simulink model "Car"  (R2024b)
settings: Solver=ode15s  StartTime=0.0  StopTime=PROFILE_LENGTH  MaxStep=300  RelTol=1e-7
values from neighbouring files (symbols this model uses):
  ACCEL_TOLERANCE = 1    [Setup.m]
  AIR_DENSITY = 1.2    [Setup.m]
  C_ROLLING_RESISTANCE = .0025    (= 0.0025)    [Setup.m]
  CONTROL_MODE = 1    [Setup.m]
  CURRENT_DATA_ECO = ECO_DATA(:, 1)    [Setup.m]
  CURRENT_DATA_POWER = POWER_DATA(:, 1)    [Setup.m]
  D_POWER = 1    [Setup.m]
  D_SPEED = 40    [Setup.m]
  DRAG_COEFFICIENT = 0.25    [Setup.m]
  DRIVER_DISPLAY_DRAW = 2.5    [Setup.m]
  FAN_DRAW = 4.8    [Setup.m]
  FORECASTED_IRRADIANCE = -5*((SOLAR_TIME_BREAKPOINTS-START_TIME).*(SOLAR_TIME_BREAKPOINTS-END_TIME) / (PROFILE_LENGTH/2)^2)    [Setup.m]
  FRONTAL_AREA = 1    [Setup.m]
  FULL_PACK_KWH = HV_PACK_VOLTAGE * HV_PACK_CAPACITY * UNIT_TO_KILO    (= 7.68)    [Setup.m]
  GRAVITY = 9.81    [Setup.m]
  HEADLIGHT_DRAW = 2    [Setup.m]
  HV_PACK_VOLTAGE = 96    [Setup.m]
  I_POWER = 1    [Setup.m]
  I_SPEED = 3    [Setup.m]
  INT_DISTANCES = COURSE_DATA(:, 8) / UNIT_TO_KILO    [Setup.m]
  INT_GRADE_ANGLE = rad2deg(atan(COURSE_DATA(:, 7)/100))    [Setup.m]
  MAX_CURRENT_ECO = max(CURRENT_DATA_ECO)    [Setup.m]
  MAX_CURRENTS_ECO = flip(CURRENT_DATA_ECO)    [Setup.m]
  MAX_CURRENTS_POWER = flip(CURRENT_DATA_POWER)    [Setup.m]
  P_POWER = 10    [Setup.m]
  P_SPEED = 25    [Setup.m]
  REGEN_ON = 0    [Setup.m]
  RPM_BREAKPOINTS_ECO = flip(RPM_DATA_ECO)    [Setup.m]
  RPM_BREAKPOINTS_POWER = flip(RPM_DATA_POWER)    [Setup.m]
  RPM_DATA_ECO = ECO_DATA(:, 3)    [Setup.m]
  RPM_DATA_POWER = POWER_DATA(:, 3)    [Setup.m]
  SECONDS_PER_HOUR = 3600    [Setup.m]
  SOLAR_TIME_BREAKPOINTS = START_TIME:900:END_TIME    [Setup.m]
  SPEED_TO_RPM = 60 / (WHEEL_DIAMETER_METERS * pi)    (= 34.1778689532)    [Setup.m]
  START_TIME = CURRENT_TIME    [Setup.m]
  STARTING_KWH = FULL_PACK_KWH * (1 - 0)    (= 7.68)    [Setup.m]
  TARGET_POWER = 700    [Setup.m]
  TARGET_SPEED = 12    [Setup.m]
  TORQUES_DATA_ECO = ECO_DATA(:, 2)    [Setup.m]
  TORQUES_DATA_POWER = POWER_DATA(:, 2) * 2.5    [Setup.m]
  TOTAL_MASS = CAR_MASS + DRIVER_MASS    (= 282.996279643)    [Setup.m]
  UNIT_TO_KILO = 1 / 1000    (= 0.001)    [Setup.m]
  WHEEL_RADIUS = WHEEL_DIAMETER_METERS / 2    (= 0.2794)    [Setup.m]
undefined symbols (not defined in the file or in its folder): density, density_elevation, distance, elevation, INT_CURRENTS, INT_TORQUES_ECO, MAX_TORQUE
libraries: slpidlib x4, simulink x1
(part 1 of 2)
settings Model: SimulationMode=accelerator  Creator=jcpetrie  LastModifiedBy=luoog
settings ModelReferenceCC: EnableRefExpFcnMdlSchedulingChecks=on
settings RTWCC: GPUComputeCapability=3.5

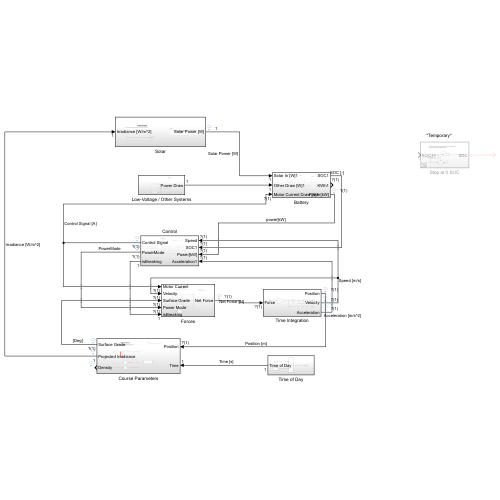
[thumbnail: Simulink's stored preview of the top-level diagram]
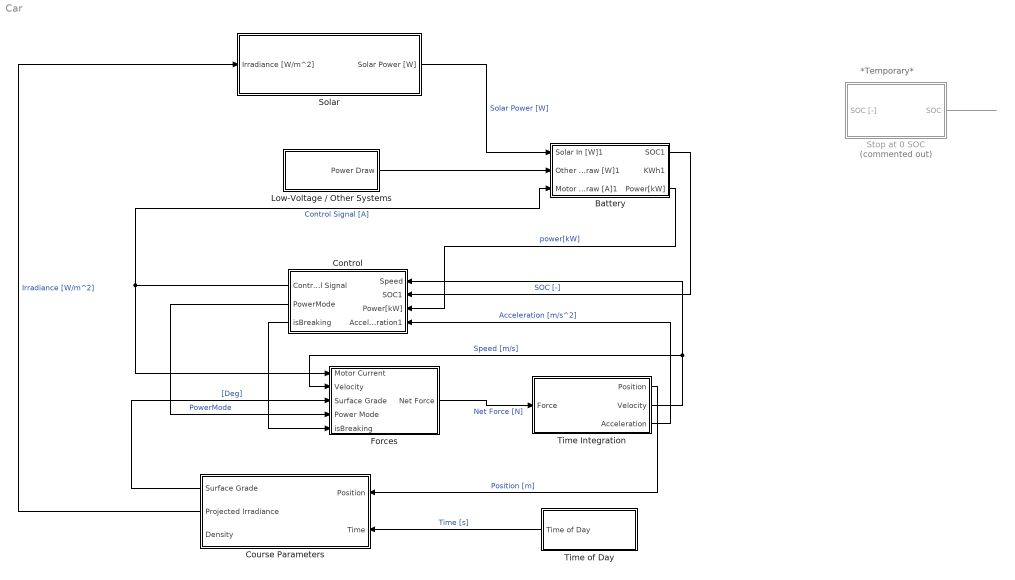
== system Car ==
  note: *Temporary*
  Battery : Subsystem
  Control : Subsystem
  Course Parameters : Subsystem
  Forces : Subsystem
  Low-Voltage / Other Systems : Subsystem
  Solar : Subsystem
  Stop at 0 SOC : Subsystem  Commented=on
  Time Integration : Subsystem
  Time of Day : Subsystem
  wires:
  Control/1(Control Signal) -> Forces/1(Motor Current), Battery/3(Motor Current Draw [A]1)  "Control Signal [A]"
  Time Integration/2(Velocity) -> Control/1(Speed), Forces/2(Velocity)  "Speed [m/s]"
  Forces/1(Net Force) -> Time Integration/1(Force)  "Net Force [N]"
  Time Integration/1(Position) -> Course Parameters/1(Position)  "Position [m]"
  Time Integration/3(Acceleration) -> Control/4(Acceleration1)  "Acceleration [m/s^2]"
  Battery/1(SOC1) -> Control/2(SOC1)  "SOC [-]"
  Course Parameters/1(Surface Grade) -> Forces/3(Surface Grade)  "[Deg]"
  Time of Day/1(Time of Day) -> Course Parameters/2(Time)  "Time [s]"
  Low-Voltage / Other Systems/1(Power Draw) -> Battery/2(Other Draw [W]1)
  Solar/1(Solar Power [W]) -> Battery/1(Solar In [W]1)  "Solar Power [W]"
  Course Parameters/2(Projected Irradiance) -> Solar/1(Irradiance [W/m^2])  "Irradiance [W/m^2]"
  Stop at 0 SOC/1(SOC) -> ?
  Control/2(PowerMode) -> Forces/4(Power Mode)  "PowerMode"
  Battery/3(Power[kW]) -> Control/3(Power[kW])  "power[kW]"
  Control/3(isBreaking) -> Forces/5(isBreaking)

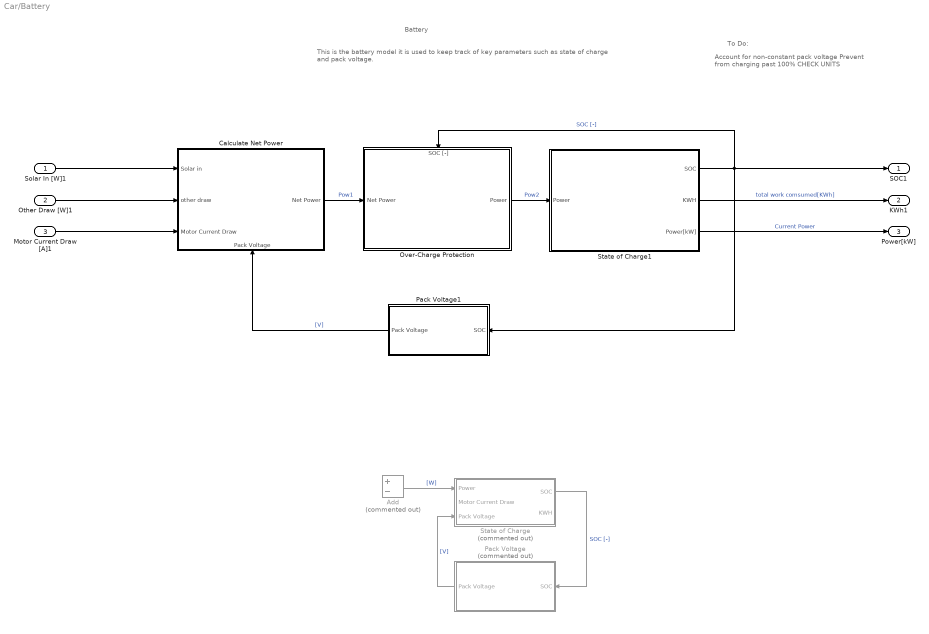
== system Car/Battery ==
  note: To Do:
  note: Battery
  note: This is the battery model it is used to keep track of key parameters such as state of charge and pack voltage.
  note: Account for non-constant pack voltage
      | Prevent from charging past 100%
      | CHECK UNITS
  Solar In [W]1 : Inport
  Other Draw [W]1 : Inport  Port=2
  Motor Current Draw [A]1 : Inport  Port=3
  Add : Sum  Commented=on  Inputs=+-
  Calculate Net Power : Subsystem
      settings: PortSchema="{\"entries\":[{\"content\":{\"sides\":[{\"content\":{\"connectorIds\":[\"In1\",\"In2\",\"In3\"]},\"type\":\"ConnectorPlacement.EquallySpacedRectSide\",\"uuid\":\"e2d2fa73-115a-40a5-bea4-fb1b26f60a86\"},{\"content\":{\"connectorIds\":[\"Out1\"],\"side\":\"RIGHT\"},\"type\":\"ConnectorPlacement.EquallySpacedRectSide\",\"uuid\":\"335f4958-33fa-4255-a87e-d106c2a4918a\"},{\"content\":{\"side\":\"TOP\"},\"type\":\"ConnectorPlacement.EquallySpacedRectSide\",\"uuid\":\"26642419-6030-44a7-8261-db287cf2270e\"},{\"content\":{\"connectorIds\":[\"In4\"],\"side\":\"BOTTOM\"},\"type\":\"ConnectorPlacement.EquallySpacedRectSide\",\"uuid\":\"d53dd7d0-088a-4c9e-b08b-c273ee7e07d3\"}]},\"type\":\"ConnectorPlacement.EquallySpacedConnector\",\"uuid\":\"42977d53-f442-47db-8063-79accecc7adb\"}],\"packageUris\":[\"http://schema.mathworks.com/mf0/Connector/R2020b\"],\"version\":\"1.0\"}"
  Over-Charge Protection : Subsystem
      settings: PortSchema="{\"entries\":[{\"content\":{\"sides\":[{\"content\":{\"connectorIds\":[\"In1\"]},\"type\":\"ConnectorPlacement.EquallySpacedRectSide\",\"uuid\":\"1fd324fe-6fd8-4ed1-a4cf-cd3bc9d77a53\"},{\"content\":{\"connectorIds\":[\"Out1\"],\"side\":\"RIGHT\"},\"type\":\"ConnectorPlacement.EquallySpacedRectSide\",\"uuid\":\"bec321c3-fba2-4d2c-8de0-ad4890ffe26d\"},{\"content\":{\"connectorIds\":[\"In2\"],\"side\":\"TOP\"},\"type\":\"ConnectorPlacement.EquallySpacedRectSide\",\"uuid\":\"f35092d8-5394-4c70-b61a-60d5076cf1ad\"}]},\"type\":\"ConnectorPlacement.EquallySpacedConnector\",\"uuid\":\"3315ea1d-8e02-4ec7-b1c7-14a34191fa6e\"}],\"packageUris\":[\"http://schema.mathworks.com/mf0/Connector/R2020b\"],\"version\":\"1.0\"}"
  Pack Voltage : Subsystem  Commented=on
  Pack Voltage1 : Subsystem
  State of Charge : Subsystem  Commented=on
  State of Charge1 : Subsystem
  SOC1 : Outport
  KWh1 : Outport  Port=2
  Power[kW] : Outport  Port=3
  wires:
  State of Charge/1(SOC) -> Pack Voltage/1(SOC)  "SOC [-]"
  Pack Voltage/1(Pack Voltage) -> State of Charge/3(Pack Voltage)  "[V]"
  Add/1 -> State of Charge/1("Power ")  "[W]"
  State of Charge1/2(KWH) -> KWh1/1  "total work comsumed[KWh]"
  Over-Charge Protection/1(Power) -> State of Charge1/1("Power ")  "Pow2"
  State of Charge1/3(Power[kW]) -> Power[kW]/1  "Current Power"
  Other Draw [W]1/1 -> Calculate Net Power/2(other draw)
  Solar In [W]1/1 -> Calculate Net Power/1(Solar in)
  Motor Current Draw [A]1/1 -> Calculate Net Power/3(Motor Current Draw)
  State of Charge1/1(SOC) -> Pack Voltage1/1(SOC), SOC1/1, Over-Charge Protection/2(SOC [-])  "SOC [-]"
  Calculate Net Power/1(Net Power) -> Over-Charge Protection/1(Net Power)  "Pow1"
  Pack Voltage1/1(Pack Voltage) -> Calculate Net Power/4(Pack Voltage)  "[V]"

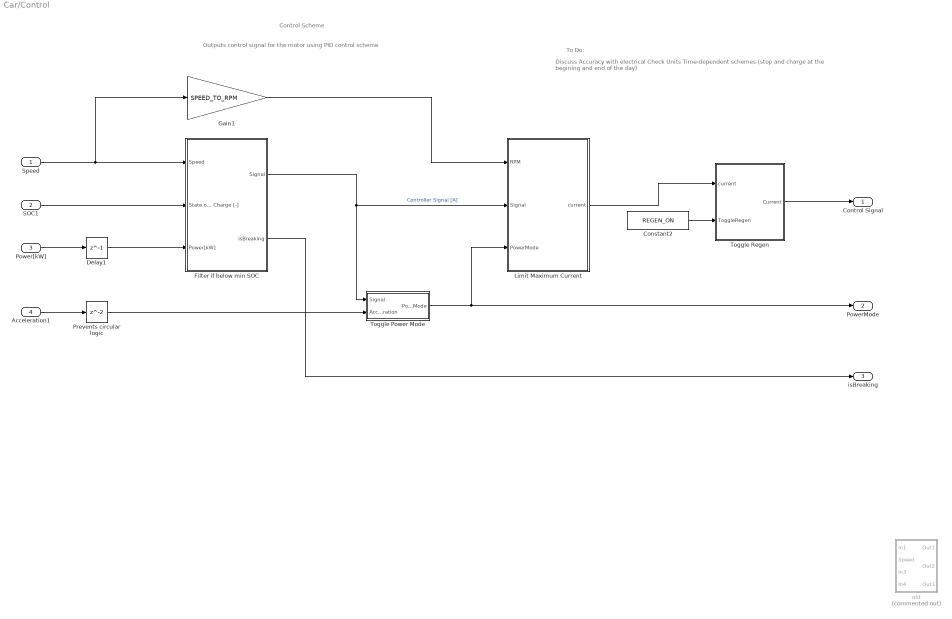
== system Car/Control ==
  note: Outputs control signal for the motor using PID control scheme
  note: To Do:
  note: Control Scheme
  note: Discuss Accuracy with electrical
      | Check Units
      | Time-dependent schemes (stop and charge at the begining and end of the day)
  Speed : Inport
  SOC1 : Inport  Port=2
  Power[kW] : Inport  Port=3
  Acceleration1 : Inport  Port=4
  Constant2 : Constant  Value=REGEN_ON
  Delay1 : Delay  DelayLength=1  SampleTime=5
  Filter if below min SOC : Subsystem
  Gain1 : Gain  Gain=SPEED_TO_RPM
  Limit Maximum Current : Subsystem
  Prevents circular logic : Delay
  Toggle Power Mode : Subsystem
  Toggle Regen : Subsystem
  old : Subsystem  Commented=on
  Control Signal : Outport
  PowerMode : Outport  Port=2
  isBreaking : Outport  Port=3
  wires:
  Toggle Power Mode/1(PowerMode) -> PowerMode/1, Limit Maximum Current/3(PowerMode)
  Limit Maximum Current/1(current) -> Toggle Regen/1(current)
  Toggle Regen/1(Current) -> Control Signal/1
  Constant2/1 -> Toggle Regen/2(ToggleRegen)
  Speed/1 -> Gain1/1, Filter if below min SOC/1(Speed)
  Prevents circular logic/1 -> Toggle Power Mode/2(Acceleration)
  SOC1/1 -> Filter if below min SOC/2(State of Charge [-])
  Filter if below min SOC/2(isBreaking) -> isBreaking/1
  Filter if below min SOC/1(Signal) -> Toggle Power Mode/1(Signal), Limit Maximum Current/2(Signal)  "Controller Signal [A]"
  Gain1/1 -> Limit Maximum Current/1(RPM)
  Power[kW]/1 -> Delay1/1
  Acceleration1/1 -> Prevents circular logic/1
  Delay1/1 -> Filter if below min SOC/3(Power[kW])

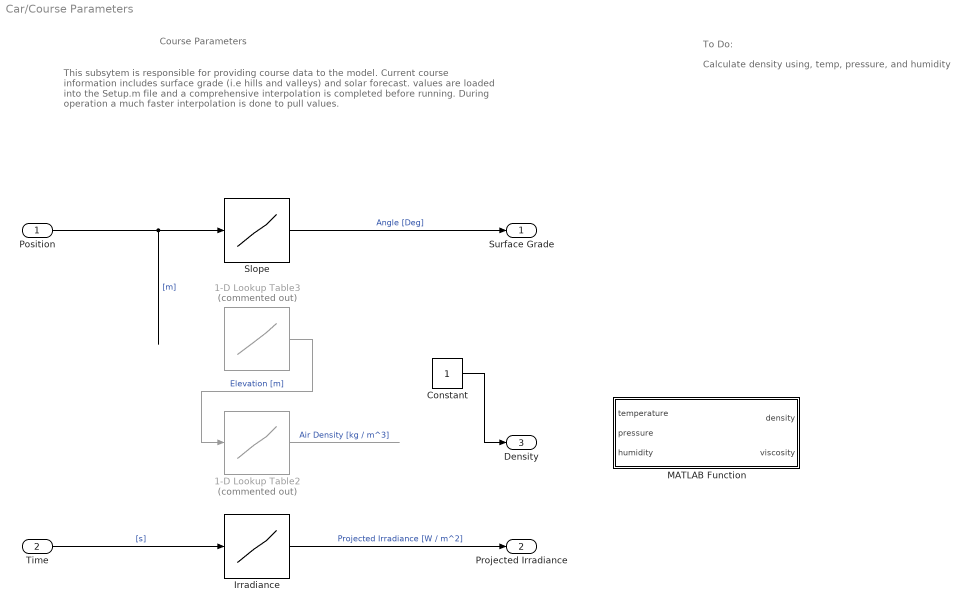
== system Car/Course Parameters ==
  note: Course Parameters
  note: This subsytem is responsible for providing course data to the model. Current course information includes surface grade (i.e hills and valleys) and solar forecast. values are loaded into the Setup.m file and a comprehensive interpolation is completed before running. During operation a much faster interpolation is done to pull values.
  note: To Do:
  note: Calculate density using, temp, pressure, and humidity
  Position : Inport
  Time : Inport  Port=2
  1-D Lookup Table2 : Lookup_n-D  Commented=on  NumberOfTableDimensions=1  BreakpointsForDimension1=density_elevation  Table=density  InternalRulePriority=Speed  RndMeth=Simplest
  1-D Lookup Table3 : Lookup_n-D  Commented=on  NumberOfTableDimensions=1  BreakpointsForDimension1=distance  Table=elevation  InternalRulePriority=Speed  RndMeth=Simplest
  Constant : Constant
  Irradiance : Lookup_n-D  NumberOfTableDimensions=1  BreakpointsForDimension1=SOLAR_TIME_BREAKPOINTS  Table=FORECASTED_IRRADIANCE  InternalRulePriority=Speed  RndMeth=Simplest
  MATLAB Function : MATLAB Function  TreatAsAtomicUnit=on
  Slope : Lookup_n-D  NumberOfTableDimensions=1  BreakpointsForDimension1=INT_DISTANCES  IndexSearchMethod=Linear search  Table=INT_GRADE_ANGLE  ExtrapMethod=Clip  UseLastTableValue=on  InternalRulePriority=Speed  RndMeth=Simplest
  Surface Grade : Outport
  Projected Irradiance : Outport  Port=2
  Density : Outport  Port=3
  wires:
  Position/1 -> Slope/1  "[m]"
  Time/1 -> Irradiance/1  "[s]"
  Slope/1 -> Surface Grade/1  "Angle [Deg]"
  Irradiance/1 -> Projected Irradiance/1  "Projected Irradiance [W / m^2]"
  1-D Lookup Table3/1 -> 1-D Lookup Table2/1  "Elevation [m]"
  1-D Lookup Table2/1 -> ?  "Air Density [kg / m^3]"
  Constant/1 -> Density/1

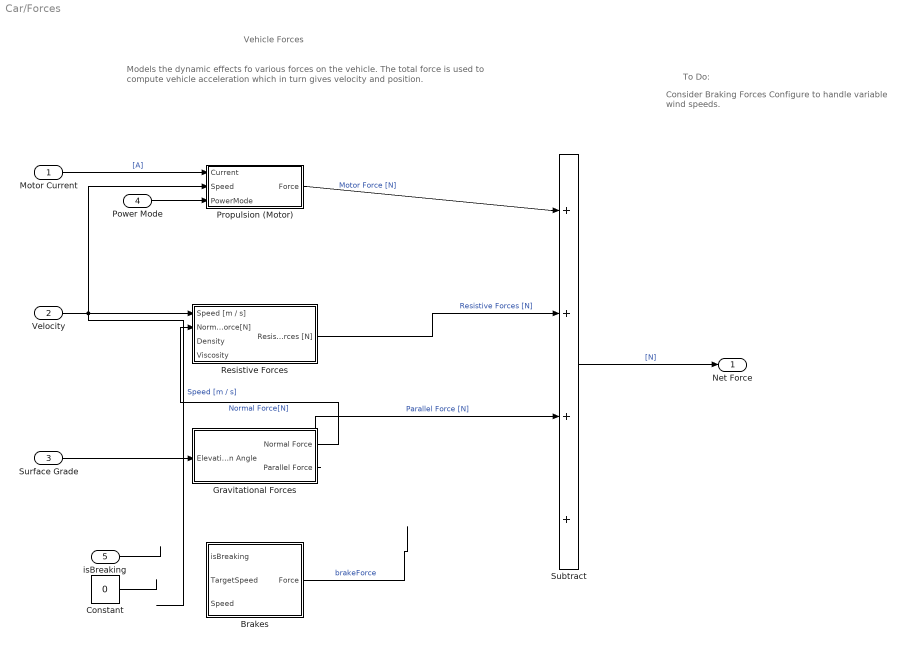
== system Car/Forces ==
  note: To Do:
  note: Vehicle Forces
  note: Models the dynamic effects fo various forces on the vehicle. The total force is used to compute vehicle acceleration which in turn gives velocity and position.
  note: Consider Braking Forces
      | Configure to handle variable wind speeds.
  Motor Current : Inport
  Velocity : Inport  Port=2
  Surface Grade : Inport  Port=3
  Power Mode : Inport  Port=4
  isBreaking : Inport  Port=5
  Brakes : Subsystem
  Constant : Constant  Value=0
  Gravitational Forces : Subsystem
  Propulsion (Motor) : Subsystem
  Resistive Forces : Subsystem
  Subtract : Sum  Inputs=+|+|++
  Net Force : Outport
  wires:
  Propulsion (Motor)/1(Force) -> Subtract/1  "Motor Force [N]"
  Subtract/1 -> Net Force/1  "[N]"
  Motor Current/1 -> Propulsion (Motor)/1(Current)  "[A]"
  Surface Grade/1 -> Gravitational Forces/1(Elevation Angle)
  Gravitational Forces/2(Parallel Force) -> Subtract/3  "Parallel Force [N]"
  Velocity/1 -> Propulsion (Motor)/2(Speed), Resistive Forces/1(Speed [m / s])  "Speed [m / s]"
  Gravitational Forces/1(Normal Force) -> Resistive Forces/2(Normal Force[N])  "Normal Force[N]"
  Resistive Forces/1(Resistive Forces [N]) -> Subtract/2  "Resistive Forces [N]"
  Power Mode/1 -> Propulsion (Motor)/3(PowerMode)
  Constant/1 -> ?
  isBreaking/1 -> ?
  Brakes/1(Force) -> ?  "brakeForce"

== system Car/Low-Voltage // Other Systems ==
  note: Lights
      | Display
      | Raspberry Pi
  Constant1 : Constant  Value=DRIVER_DISPLAY_DRAW
  Constant2 : Constant  Value=HEADLIGHT_DRAW
  Fans : Constant  Value=FAN_DRAW
  Sum : Sum  Inputs=+++
  Power Draw : Outport
  wires:
  Constant1/1 -> Sum/2  "[W]"
  Sum/1 -> Power Draw/1  "[W]"
  Fans/1 -> Sum/1  "[W]"
  Constant2/1 -> Sum/3  "[W]"

== system Car/Solar ==
  note: Remove constant power out
      | Replace with conversion function based on experimental data which converts irradiance to power
  note: Converts expected irradiance to solar out. Based on testing data.
  note: Solar Power
  note: To Do:
  Irradiance [W/m^2] : Inport
  Solar Power [W] : Outport
  wires:
  Irradiance [W/m^2]/1 -> Solar Power [W]/1

== system Car/Stop at 0 SOC ==
  note: This block is a temporary fix meant to adress issues that occor when the car attempts to draw power when the battery is empty.
  SOC [-] : Inport
  If : If
  If Action Subsystem : Subsystem  TreatAsAtomicUnit=on
  If Action Subsystem1 : Subsystem  TreatAsAtomicUnit=on
  Stop Simulation : Stop
  SOC : Outport
  wires:
  If/1 -> If Action Subsystem/Action
  SOC [-]/1 -> If Action Subsystem1/1(SOC), If Action Subsystem/1(SOC), If/1
  If Action Subsystem1/1(Out1) -> Stop Simulation/1
  If/2 -> If Action Subsystem1/Action
  If Action Subsystem/1(Out1) -> SOC/1

== system Car/Time Integration ==
  Force : Inport
  Gain : Gain  Gain=1 / TOTAL_MASS
  Integrator : Integrator
  Integrator1 : Integrator
  Position : Outport
  Velocity : Outport  Port=2
  Acceleration : Outport  Port=3
  wires:
  Gain/1 -> Acceleration/1, Integrator/1  "Acceleration [m/s^2]"
  Integrator/1 -> Velocity/1, Integrator1/1  "Velocity [m/s]"
  Force/1 -> Gain/1  "[N]"
  Integrator1/1 -> Position/1  "Position [m]"

== system Car/Time of Day ==
  Add : Sum
  Clock : Clock
  Constant : Constant  Value=START_TIME
  Time of Day : Outport
  wires:
  Add/1 -> Time of Day/1  "Time of Day [s]"
  Clock/1 -> Add/1  "Simulation Time [s]"
  Constant/1 -> Add/2  "Start time of day [s]"

== system Car/Battery/Calculate Net Power ==
  Solar in : Inport
  other draw : Inport  Port=2
  Motor Current Draw : Inport  Port=3
  Pack Voltage : Inport  Port=4
  Plus : Sum  Inputs=+--
  Product : Product  Inputs=**
  Net Power : Outport
  wires:
  Product/1 -> Plus/3  "[W]"
  Plus/1 -> Net Power/1
  Motor Current Draw/1 -> Product/1  "[A]"
  Pack Voltage/1 -> Product/2  "[V]"
  other draw/1 -> Plus/2
  Solar in/1 -> Plus/1

== system Car/Battery/Over-Charge Protection ==
  Net Power : Inport
  SOC [-] : Inport  Port=2
  Charged status : Merge
  Fully charged : Subsystem  TreatAsAtomicUnit=on
  Not fully charged : Subsystem  TreatAsAtomicUnit=on
  Overcharge Prevention : If  IfExpression=u1 >=MAX_SOC  ZeroCross=off
  Power : Outport
  wires:
  Net Power/1 -> Fully charged/1(Net Power), Not fully charged/1(Solar In [W])
  Overcharge Prevention/1 -> Fully charged/Action
  Fully charged/1(Out1) -> Charged status/1
  Not fully charged/1(Out1) -> Charged status/2
  Charged status/1 -> Power/1  "Net Power"
  SOC [-]/1 -> Overcharge Prevention/1
  Overcharge Prevention/2 -> Not fully charged/Action

== system Car/Battery/Pack Voltage ==
  note: Battery Voltage
  note: Outputs the Voltage of the battery given the state of charge
  note: To Do:
  note: Get voltage curve from battery, implment non constant behavior.
  SOC : Inport
  Constant : Constant  Value=HV_PACK_VOLTAGE
  Pack Voltage : Outport
  wires:
  SOC/1 -> ?
  Constant/1 -> Pack Voltage/1  "[V]"

== system Car/Battery/Pack Voltage1 ==
  note: Battery Voltage
  note: Outputs the Voltage of the battery given the state of charge
  note: To Do:
  note: Get voltage curve from battery, implment non constant behavior.
  SOC : Inport
  Constant : Constant  Value=HV_PACK_VOLTAGE
  Pack Voltage : Outport
  wires:
  SOC/1 -> ?
  Constant/1 -> Pack Voltage/1  "[V]"

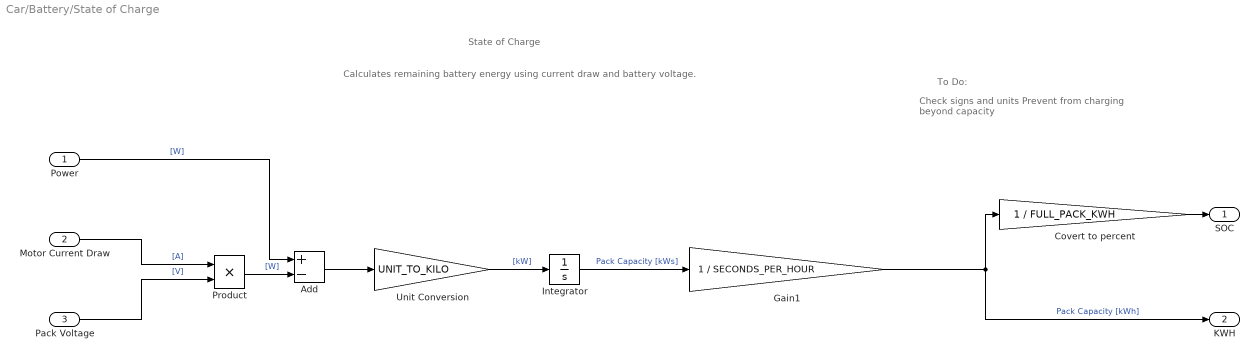
== system Car/Battery/State of Charge ==
  note: State of Charge
  note: Check signs and units
      | Prevent from charging beyond capacity
  note: To Do:
  note: Calculates remaining battery energy using current draw and battery voltage.
  "Power " : Inport
  Motor Current Draw : Inport  Port=2
  Pack Voltage : Inport  Port=3
  Add : Sum  Inputs=+-
  Covert to percent : Gain  Gain=1 / FULL_PACK_KWH
  Gain1 : Gain  Gain=1 / SECONDS_PER_HOUR
  Integrator : Integrator  InitialCondition=STARTING_KWH * SECONDS_PER_HOUR
  Product : Product  Inputs=**
  Unit Conversion : Gain  Gain=UNIT_TO_KILO
  SOC : Outport
  KWH : Outport  Port=2
  wires:
  Integrator/1 -> Gain1/1  "Pack Capacity [kWs]"
  Covert to percent/1 -> SOC/1
  Pack Voltage/1 -> Product/2  "[V]"
  Product/1 -> Add/2  "[W]"
  Unit Conversion/1 -> Integrator/1  "[kW]"
  Motor Current Draw/1 -> Product/1  "[A]"
  Gain1/1 -> KWH/1, Covert to percent/1  "Pack Capacity [kWh]"
  "Power "/1 -> Add/1  "[W]"
  Add/1 -> Unit Conversion/1

== system Car/Battery/State of Charge1 ==
  note: State of Charge
  note: Check signs and units
      | Prevent from charging beyond capacity
  note: To Do:
  note: Calculates remaining battery energy using current draw and battery voltage.
  "Power " : Inport
  Covert to percent : Gain  Gain=1 / FULL_PACK_KWH
  Gain1 : Gain  Gain=1 / SECONDS_PER_HOUR
  Integrator : Integrator  InitialCondition=STARTING_KWH * SECONDS_PER_HOUR
  Unit Conversion : Gain  Gain=UNIT_TO_KILO
  SOC : Outport
  KWH : Outport  Port=2
  Power[kW] : Outport  Port=3
  wires:
  Integrator/1 -> Gain1/1  "Pack Capacity [kWs]"
  Covert to percent/1 -> SOC/1
  Unit Conversion/1 -> Power[kW]/1, Integrator/1  "[kW]"
  Gain1/1 -> KWH/1, Covert to percent/1  "Pack Capacity [kWh]"
  "Power "/1 -> Unit Conversion/1  "[W]"

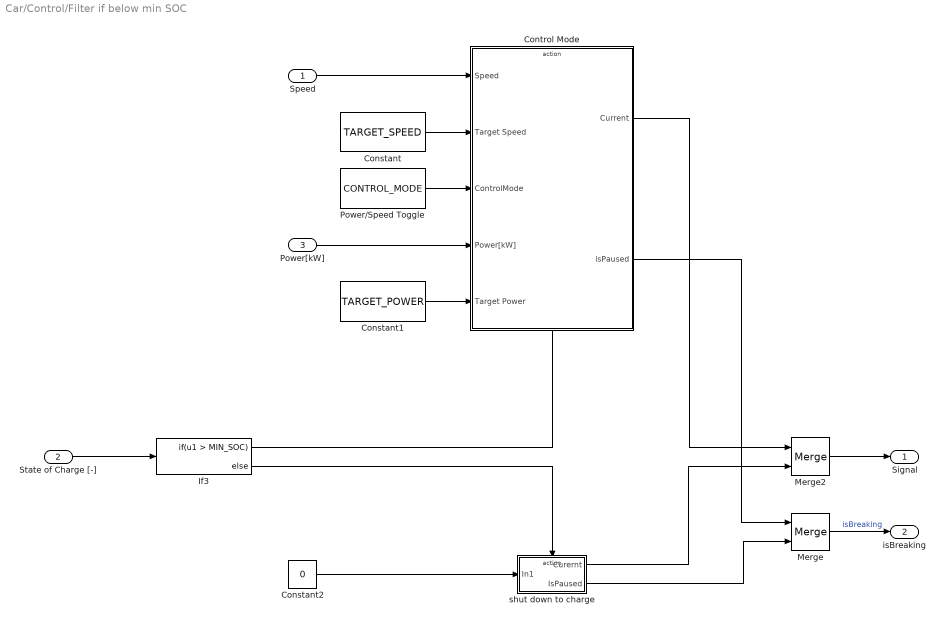
== system Car/Control/Filter if below min SOC ==
  Speed : Inport
  State of Charge [-] : Inport  Port=2
  Power[kW] : Inport  Port=3
  Constant : Constant  Value=TARGET_SPEED
  Constant1 : Constant  Value=TARGET_POWER
  Constant2 : Constant  Value=0
  Control Mode : Subsystem  TreatAsAtomicUnit=on
  If3 : If  IfExpression=u1 > MIN_SOC  ZeroCross=off
  Merge : Merge
  Merge2 : Merge
  Power/Speed Toggle : Constant  Value=CONTROL_MODE
  shut down to charge : Subsystem  TreatAsAtomicUnit=on
  Signal : Outport
  isBreaking : Outport  Port=2
  wires:
  shut down to charge/1(Curernt) -> Merge2/2
  Merge2/1 -> Signal/1
  If3/2 -> shut down to charge/Action
  If3/1 -> Control Mode/Action
  Constant2/1 -> shut down to charge/1(In1)
  State of Charge [-]/1 -> If3/1
  Control Mode/1(Current) -> Merge2/1
  Speed/1 -> Control Mode/1(Speed)
  Power/Speed Toggle/1 -> Control Mode/3(ControlMode)
  Power[kW]/1 -> Control Mode/4(Power[kW])
  Constant/1 -> Control Mode/2(Target Speed)
  Constant1/1 -> Control Mode/5(Target Power)
  Control Mode/2(isPaused) -> Merge/1
  Merge/1 -> isBreaking/1  "isBreaking"
  shut down to charge/2(IsPaused) -> Merge/2

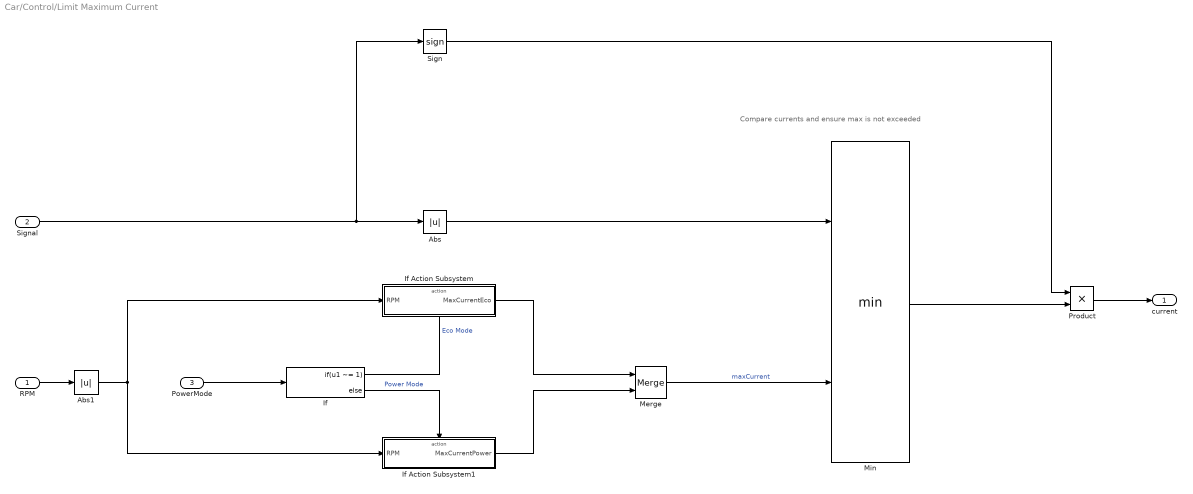
== system Car/Control/Limit Maximum Current ==
  note: Compare currents and ensure max is not exceeded
  RPM : Inport
  Signal : Inport  Port=2
  PowerMode : Inport  Port=3
  Abs : Abs  ZeroCross=off  SaturateOnIntegerOverflow=off
  Abs1 : Abs  ZeroCross=off  SaturateOnIntegerOverflow=off
  If : If  IfExpression=u1 ~= 1
  If Action Subsystem : Subsystem  TreatAsAtomicUnit=on
  If Action Subsystem1 : Subsystem  TreatAsAtomicUnit=on
  Merge : Merge
  Min : MinMax  Inputs=2
  Product : Product
  Sign : Signum  ZeroCross=off
  current : Outport
  wires:
  PowerMode/1 -> If/1
  If/1 -> If Action Subsystem/Action  "Eco Mode"
  If/2 -> If Action Subsystem1/Action  "Power Mode"
  RPM/1 -> Abs1/1
  If Action Subsystem/1(MaxCurrentEco) -> Merge/1
  If Action Subsystem1/1(MaxCurrentPower) -> Merge/2
  Merge/1 -> Min/2  "maxCurrent"
  Signal/1 -> Sign/1, Abs/1
  Abs/1 -> Min/1
  Min/1 -> Product/2
  Sign/1 -> Product/1
  Product/1 -> current/1
  Abs1/1 -> If Action Subsystem1/1(RPM), If Action Subsystem/1(RPM)

== system Car/Control/Toggle Power Mode ==
  note: Eco/Power Mode
  note: Decides when to change the car to be in power mode.
  Signal : Inport
  Acceleration : Inport  Port=2
  AND : Logic  IconShape=distinctive  AllPortsSameDT=off  OutDataTypeStr=boolean
  Constant : Constant  Value=MAX_CURRENT_ECO
  Constant1 : Constant  Value=ACCEL_TOLERANCE
  Relational Operator : RelationalOperator  OutDataTypeStr=boolean  RndMeth=Simplest  InputSameDT=off
  Relational Operator1 : RelationalOperator  Operator=<=  OutDataTypeStr=boolean  RndMeth=Simplest  InputSameDT=off
  Zero-Order Hold : ZeroOrderHold
  PowerMode : Outport
  wires:
  Relational Operator/1 -> AND/1
  Signal/1 -> Relational Operator/1  "signal"
  Constant/1 -> Relational Operator/2
  Relational Operator1/1 -> AND/2
  Acceleration/1 -> Relational Operator1/1  "accleration"
  AND/1 -> Zero-Order Hold/1
  Constant1/1 -> Relational Operator1/2
  Zero-Order Hold/1 -> PowerMode/1

== system Car/Control/Toggle Regen ==
  current : Inport
  ToggleRegen : Inport  Port=2
  Allow Current : Subsystem  TreatAsAtomicUnit=on
  Constant : Constant  Value=0
  If : If  NumInputs=2  IfExpression=~u1 & u2<0
  Merge : Merge
  Prevent Regen : Subsystem  TreatAsAtomicUnit=on
  Current : Outport
  wires:
  If/1 -> Prevent Regen/Action
  If/2 -> Allow Current/Action
  current/1 -> If/2, Allow Current/1(current)
  Merge/1 -> Current/1
  Prevent Regen/1(Out1) -> Merge/1
  Allow Current/1(Out1) -> Merge/2
  ToggleRegen/1 -> If/1  "RegenOn"
  Constant/1 -> Prevent Regen/1(current)

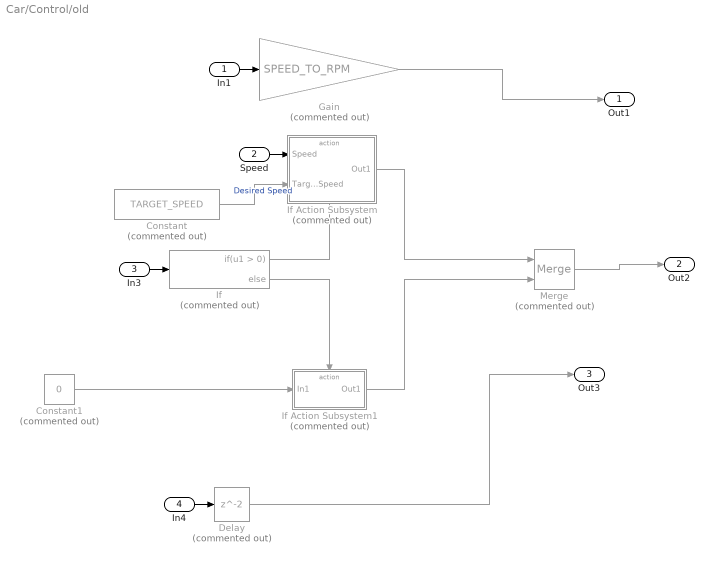
== system Car/Control/old ==
  In1 : Inport
  Speed : Inport  Port=2
  In3 : Inport  Port=3
  In4 : Inport  Port=4
  Constant : Constant  Commented=on  Value=TARGET_SPEED
  Constant1 : Constant  Commented=on  Value=0
  Delay : Delay  Commented=on
  Gain : Gain  Commented=on  Gain=SPEED_TO_RPM
  If : If  Commented=on
  If Action Subsystem : Subsystem  Commented=on  TreatAsAtomicUnit=on
  If Action Subsystem1 : Subsystem  Commented=on  TreatAsAtomicUnit=on
  Merge : Merge  Commented=on
  Out1 : Outport
  Out2 : Outport  Port=2
  Out3 : Outport  Port=3
  wires:
  Constant1/1 -> If Action Subsystem1/1(In1)
  If/2 -> If Action Subsystem1/Action
  If Action Subsystem/1(Out1) -> Merge/1
  In1/1 -> Gain/1
  If/1 -> If Action Subsystem/Action
  If Action Subsystem1/1(Out1) -> Merge/2
  Gain/1 -> Out1/1
  Constant/1 -> If Action Subsystem/2(Target Speed)  "Desired Speed"
  Merge/1 -> Out2/1
  Delay/1 -> Out3/1
  Speed/1 -> If Action Subsystem/1(Speed)
  In3/1 -> If/1
  In4/1 -> Delay/1

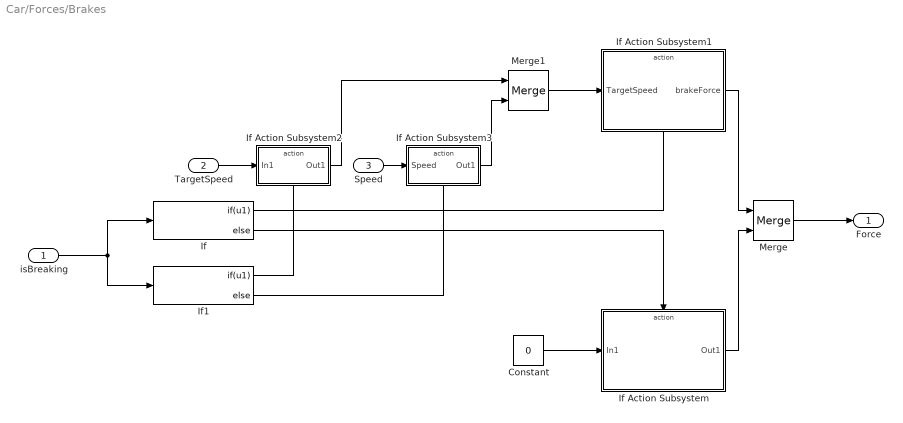
== system Car/Forces/Brakes ==
  isBreaking : Inport
  TargetSpeed : Inport  Port=2
  Speed : Inport  Port=3
  Constant : Constant  Value=0
  If : If  IfExpression=u1
  If Action Subsystem : Subsystem  TreatAsAtomicUnit=on
  If Action Subsystem1 : Subsystem  TreatAsAtomicUnit=on
  If Action Subsystem2 : Subsystem  TreatAsAtomicUnit=on
  If Action Subsystem3 : Subsystem  TreatAsAtomicUnit=on
  If1 : If  IfExpression=u1
  Merge : Merge
  Merge1 : Merge
  Force : Outport
  wires:
  isBreaking/1 -> If/1, If1/1
  If/1 -> If Action Subsystem1/Action
  If/2 -> If Action Subsystem/Action
  Merge/1 -> Force/1
  If Action Subsystem1/1(brakeForce) -> Merge/1
  If Action Subsystem/1(Out1) -> Merge/2
  Constant/1 -> If Action Subsystem/1(In1)
  TargetSpeed/1 -> If Action Subsystem2/1(In1)
  Speed/1 -> If Action Subsystem3/1(Speed)
  If Action Subsystem2/1(Out1) -> Merge1/1
  If Action Subsystem3/1(Out1) -> Merge1/2
  Merge1/1 -> If Action Subsystem1/1(TargetSpeed)
  If1/1 -> If Action Subsystem2/Action
  If1/2 -> If Action Subsystem3/Action

== system Car/Forces/Gravitational Forces ==
  note: To Do:
  note: Gravitational Forces
  note: When oparting on surfaces that aren't flat, the vehicle will expereince differing forces acting on the normal to the ground, affecting frictional losses, and parallel to the ground which can act as a hinderenace or boost depending on if it is climbing or "falling".
  Elevation Angle : Inport
  Cos : Trigonometry  Operator=cos
  Gain : Gain  Gain=TOTAL_MASS * GRAVITY
  Gain1 : Gain  Gain=TOTAL_MASS * GRAVITY
  Gain2 : Gain  Gain=-1
  Gain3 : Gain  Gain=pi/180
  Sin : Trigonometry
  Normal Force : Outport
  Parallel Force : Outport  Port=2
  wires:
  Elevation Angle/1 -> Gain3/1
  Cos/1 -> Gain/1
  Gain/1 -> Normal Force/1
  Sin/1 -> Gain1/1
  Gain1/1 -> Gain2/1
  Gain2/1 -> Parallel Force/1
  Gain3/1 -> Sin/1, Cos/1

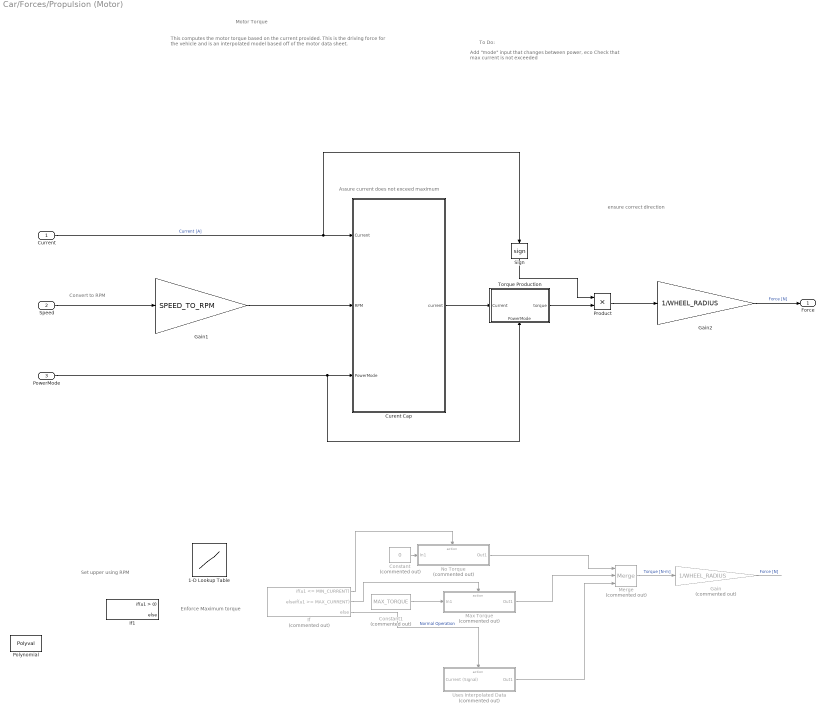
== system Car/Forces/Propulsion (Motor) ==
  note: ensure correct direction
  note: Assure current does not exceed maximum
  note: Enforce Maximum torque
  note: Set upper using RPM
  note: Convert to RPM
  note: Add "mode" input that changes between power, eco
      | Check that max current is not exceeded
  note: Motor Torque
  note: To Do:
  note: This computes the motor torque based on the current provided. This is the driving force for the vehicle and is an interpolated model based off of the motor data sheet.
  Current : Inport
  Speed : Inport  Port=2
  PowerMode : Inport  Port=3
  1-D Lookup Table : Lookup_n-D  NumberOfTableDimensions=1  BreakpointsForDimension1=[-5:5]  Table=tanh([-5:5])  InternalRulePriority=Speed  RndMeth=Simplest
  Constant : Constant  Commented=on  Value=0
  Constant1 : Constant  Commented=on  Value=MAX_TORQUE
  Curent Cap : Subsystem
  Gain : Gain  Commented=on  Gain=1/WHEEL_RADIUS
  Gain1 : Gain  Gain=SPEED_TO_RPM
  Gain2 : Gain  Gain=1/WHEEL_RADIUS
  If : If  Commented=on  IfExpression=u1 <= MIN_CURRENT  ElseIfExpressions=u1 >= MAX_CURRENT
  If1 : If
  Max Torque : Subsystem  Commented=on  TreatAsAtomicUnit=on
  Merge : Merge  Commented=on  Inputs=3
  No Torque : Subsystem  Commented=on  TreatAsAtomicUnit=on
  Polynomial : Polyval  Coefs=[ +2.081618890e-019, -1.441693666e-014, +4.719686976e-010, -8.536869453e-006, +1.621573104e-001, -8.087801117e+001 ]
  Product : Product
  Sign : Signum  ZeroCross=off
  Torque Production : Subsystem
      settings: PortSchema="{\"entries\":[{\"content\":{\"sides\":[{\"content\":{\"connectorIds\":[\"In1\"]},\"type\":\"ConnectorPlacement.EquallySpacedRectSide\",\"uuid\":\"611da849-a11b-4f2d-83b9-7ce03da94254\"},{\"content\":{\"connectorIds\":[\"Out1\"],\"side\":\"RIGHT\"},\"type\":\"ConnectorPlacement.EquallySpacedRectSide\",\"uuid\":\"6c8d5a93-87a1-407e-8b13-ad17147d051f\"},{\"content\":{\"side\":\"TOP\"},\"type\":\"ConnectorPlacement.EquallySpacedRectSide\",\"uuid\":\"47651826-5648-48f2-a524-328e0450a778\"},{\"content\":{\"connectorIds\":[\"In2\"],\"side\":\"BOTTOM\"},\"type\":\"ConnectorPlacement.EquallySpacedRectSide\",\"uuid\":\"187a6d4c-cc7b-4f39-a2d5-b40b5f6747ca\"}]},\"type\":\"ConnectorPlacement.EquallySpacedConnector\",\"uuid\":\"fe5b8080-d1e2-4c15-97fd-d52d82a06f20\"}],\"packageUris\":[\"http://schema.mathworks.com/mf0/Connector/R2020b\"],\"version\":\"1.0\"}"
  Uses Interpolated Data : Subsystem  Commented=on  TreatAsAtomicUnit=on
  Force : Outport
  wires:
  Current/1 -> Sign/1, Curent Cap/1(Current)  "Current [A]"
  Constant/1 -> No Torque/1(In1)
  If/1 -> No Torque/Action
  If/2 -> Max Torque/Action
  Uses Interpolated Data/1(Out1) -> Merge/3
  No Torque/1(Out1) -> Merge/1
  Merge/1 -> Gain/1  "Torque [N-m]"
  If/3 -> Uses Interpolated Data/Action  "Normal Operation"
  Constant1/1 -> Max Torque/1(In1)
  Max Torque/1(Out1) -> Merge/2
  Gain/1 -> ?  "Force [N]"
  Speed/1 -> Gain1/1
  PowerMode/1 -> Curent Cap/3(PowerMode), Torque Production/2(PowerMode)
  Gain1/1 -> Curent Cap/2(RPM)
  Curent Cap/1(current) -> Torque Production/1(Current)
  Sign/1 -> Product/1
  Torque Production/1(torque) -> Product/2
  Product/1 -> Gain2/1
  Gain2/1 -> Force/1  "Force [N]"

== system Car/Forces/Resistive Forces ==
  note: Flip direction if moving backwards
  note: Resistive Forces
  note: Uses velocity of the vehicle to calculate the force opposing motion.
      |
      | NOTE: These forces (particularily drag) will NOT simply change sign when going backwards. However they will be modeled that way because it is easy and currently not worth the effort to model accurately since these are not condition that we expect to drive the car in.
  Speed [m / s] : Inport
  Normal Force[N] : Inport  Port=2
  Density : Inport  Port=3
  Viscosity : Inport  Port=4
  Add : Sum
  Drag : Subsystem
  Gain : Gain  Gain=-1
  Product : Product
  Rolling Resistance : Subsystem
  Sign : Signum  ZeroCross=off
  Resistive Forces [N] : Outport
  wires:
  Speed [m / s]/1 -> Drag/1(Velocity), Rolling Resistance/1(Velocity), Sign/1
  Product/1 -> Resistive Forces [N]/1
  Rolling Resistance/1(Rolling Resistance) -> Add/2  "Rolling Resistance [N]"
  Drag/1(Drag Force) -> Add/1  "Drag Force [N]"
  Add/1 -> Product/2
  Normal Force[N]/1 -> Rolling Resistance/2(Normal Force)
  Sign/1 -> Gain/1
  Gain/1 -> Product/1

== system Car/Stop at 0 SOC/If Action Subsystem ==
  SOC : Inport
  Action Port : ActionPort  ActionPortLabel=if(u1 > 0)
  Out1 : Outport
  wires:
  SOC/1 -> Out1/1

== system Car/Stop at 0 SOC/If Action Subsystem1 ==
  SOC : Inport
  Action Port : ActionPort  ActionPortLabel=else
  Out1 : Outport
  wires:
  SOC/1 -> Out1/1

== system Car/Battery/Over-Charge Protection/Fully charged ==
  Net Power : Inport
  Action Port : ActionPort  ActionPortLabel=if(u1 >=MAX_SOC)
  IsNegative : simulink/Logic and Bit Operations/Compare To Zero  relop=<  OutDataTypeStr=boolean
      settings: LibrarySourceBlock=|
      | simulink/Quick Insert/Logic and Bit
      | Operations/IsNegative
  Product : Product
  Out1 : Outport
  wires:
  Net Power/1 -> IsNegative/1, Product/2  "Pow1"
  IsNegative/1 -> Product/1
  Product/1 -> Out1/1  "pow2"

== system Car/Battery/Over-Charge Protection/Not fully charged ==
  Solar In [W] : Inport
  Action Port : ActionPort  ActionPortLabel=else
  Out1 : Outport
  wires:
  Solar In [W]/1 -> Out1/1

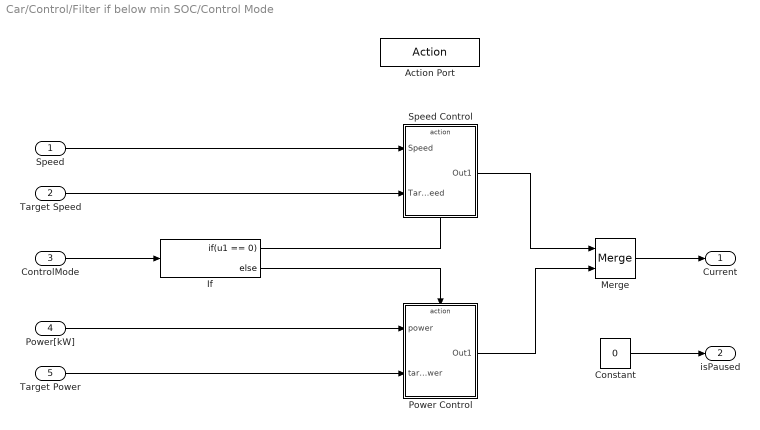
== system Car/Control/Filter if below min SOC/Control Mode ==
  Speed : Inport
  Target Speed : Inport  Port=2
  ControlMode : Inport  Port=3
  Power[kW] : Inport  Port=4
  Target Power : Inport  Port=5
  Action Port : ActionPort  ActionPortLabel=if(u1 > MIN_SOC)
  Constant : Constant  Value=0
  If : If  IfExpression=u1 == 0
  Merge : Merge
  Power Control : Subsystem  TreatAsAtomicUnit=on
  Speed Control : Subsystem  TreatAsAtomicUnit=on
  Current : Outport
  isPaused : Outport  Port=2
  wires:
  If/1 -> Speed Control/Action
  If/2 -> Power Control/Action
  Power[kW]/1 -> Power Control/1(power)
  ControlMode/1 -> If/1
  Speed/1 -> Speed Control/1(Speed)
  Target Speed/1 -> Speed Control/2(Target Speed)
  Speed Control/1(Out1) -> Merge/1
  Power Control/1(Out1) -> Merge/2
  Target Power/1 -> Power Control/2(target power)
  Merge/1 -> Current/1
  Constant/1 -> isPaused/1

== system Car/Control/Filter if below min SOC/shut down to charge ==
  In1 : Inport
  Action Port : ActionPort  ActionPortLabel=else
  Constant : Constant
  Curernt : Outport
  IsPaused : Outport  Port=2
  wires:
  In1/1 -> Curernt/1
  Constant/1 -> IsPaused/1

== system Car/Control/Limit Maximum Current/If Action Subsystem ==
  note: Eco Mode
  RPM : Inport
  Action Port : ActionPort  ActionPortLabel=if(u1 ~= 1)
  1-D Lookup Table : Lookup_n-D  NumberOfTableDimensions=1  BreakpointsForDimension1=RPM_BREAKPOINTS_ECO  IndexSearchMethod=Linear search  Table=MAX_CURRENTS_ECO  ExtrapMethod=Clip  InternalRulePriority=Speed  RndMeth=Simplest
  If : If  Commented=on  IfExpression=u1 > MAX_RPM_ECO
  If Action Subsystem : Subsystem  Commented=on  TreatAsAtomicUnit=on
  If Action Subsystem1 : Subsystem  Commented=on  TreatAsAtomicUnit=on
  Merge : Merge  Commented=on
  MaxCurrentEco : Outport
  wires:
  If/1 -> If Action Subsystem/Action  "OutOfRange"
  If/2 -> If Action Subsystem1/Action  "inRange"
  Merge/1 -> ?  "MaxCurrentEco"
  If Action Subsystem1/1(MaxCurrentEco) -> Merge/2
  If Action Subsystem/1(Out1) -> Merge/1
  1-D Lookup Table/1 -> MaxCurrentEco/1
  RPM/1 -> 1-D Lookup Table/1

== system Car/Control/Limit Maximum Current/If Action Subsystem1 ==
  note: Power Mode
  RPM : Inport
  Action Port : ActionPort  ActionPortLabel=else
  1-D Lookup Table : Lookup_n-D  NumberOfTableDimensions=1  BreakpointsForDimension1=RPM_BREAKPOINTS_POWER  Table=MAX_CURRENTS_POWER  ExtrapMethod=Clip  InternalRulePriority=Speed  RndMeth=Simplest
  If : If  Commented=on  IfExpression=u1 > MAX_RPM_POWER
  If Action Subsystem : Subsystem  Commented=on  TreatAsAtomicUnit=on
  If Action Subsystem1 : Subsystem  Commented=on  TreatAsAtomicUnit=on
  Merge : Merge  Commented=on
  MaxCurrentPower : Outport
  wires:
  If Action Subsystem/1(Out1) -> Merge/1
  If Action Subsystem1/1(MaxCurrentEco) -> Merge/2
  If/1 -> If Action Subsystem/Action  "OutOfRange"
  Merge/1 -> ?  "MaxCurrentPower"
  If/2 -> If Action Subsystem1/Action  "inRange"
  RPM/1 -> 1-D Lookup Table/1
  1-D Lookup Table/1 -> MaxCurrentPower/1

== system Car/Control/Toggle Regen/Allow Current ==
  current : Inport
  Action Port : ActionPort  ActionPortLabel=else
  Out1 : Outport
  wires:
  current/1 -> Out1/1

== system Car/Control/Toggle Regen/Prevent Regen ==
  current : Inport
  Action Port : ActionPort  ActionPortLabel=if(~u1 & u2<0)
  Out1 : Outport
  wires:
  current/1 -> Out1/1

== system Car/Control/old/If Action Subsystem ==
  Speed : Inport
  Target Speed : Inport  Port=2
  Action Port : ActionPort  ActionPortLabel=if(u1 > 0)
  PID Controller : slpidlib/PID Controller  Controller=PID  Form=Parallel  TimeDomain=Continuous-time  UseExternalTs=off  SampleTime=-1  IntegratorMethod=Forward Euler  FilterMethod=Forward Euler  ControllerParametersSource=internal  P=2.5  I=0.1  UseKiTs=off  D=0  N=100  UseFilter=on  TunerSelectOption=Transfer Function Based (PID Tuner App)  InitialConditionSource=internal  InitialConditionForIntegrator=0  InitialConditionForFilter=0  DifferentiatorICPrevScaledInput=0  ExternalReset=none  TrackingMode=off  Kt=1  LimitOutput=off  SatLimitsSource=internal  UpperSaturationLimit=inf  LowerSaturationLimit=-inf  LinearizeAsGain=on  AntiWindupMode=none  Kb=1  LimitIntegrator=off  UpperIntegratorSaturationLimit=inf  LowerIntegratorSaturationLimit=-inf  POutMin=[]  POutMax=[]  IOutMin=[]  IOutMax=[]  DOutMin=[]  DOutMax=[]  NOutMin=[]  NOutMax=[]  SumOutMin=[]  SumOutMax=[]  SaturationOutMin=[]  SaturationOutMax=[]  PParamMin=[]  PParamMax=[]  IParamMin=[]  IParamMax=[]  DParamMin=[]  DParamMax=[]  NParamMin=[]  NParamMax=[]  KbParamMin=[]  KbParamMax=[]  KtParamMin=[]  KtParamMax=[]  KbOutMin=[]  KbOutMax=[]  KtOutMin=[]  KtOutMax=[]  IntegratorOutMin=[]  IntegratorOutMax=[]  FilterOutMin=[]  FilterOutMax=[]  SumI1OutMin=[]  SumI1OutMax=[]  SumI2OutMin=[]  SumI2OutMax=[]  SumI3OutMin=[]  SumI3OutMax=[]  SumI4OutMin=[]  SumI4OutMax=[]  SumDOutMin=[]  SumDOutMax=[]  DifferentiatorOutMin=[]  DifferentiatorOutMax=[]  FilterDiffOutCoefMin=[]  FilterDiffOutCoefMax=[]  ReciprocalOutMin=[]  ReciprocalOutMax=[]  SumDenOutMin=[]  SumDenOutMax=[]  SumNumOutMin=[]  SumNumOutMax=[]  DivideOutMin=[]  DivideOutMax=[]  UdiffTsProdOutMin=[]  UdiffTsProdOutMax=[]  NTsProdOutMin=[]  NTsProdOutMax=[]  UintegralTsProdOutMin=[]  UintegralTsProdOutMax=[]  UngainTsProdOutMin=[]  UngainTsProdOutMax=[]  ClampingZeroOutDataTypeStr=Inherit: Inherit via back propagation  ClampingZeroOutMin=[]  ClampingZeroOutMax=[]  FilterDenConstantOutDataTypeStr=Inherit: Inherit via back propagation  FilterDenConstantOutMin=[]  FilterDenConstantOutMax=[]  PCopyOutDataTypeStr=Inherit: Inherit via back propagation  PCopyOutMin=[]  PCopyOutMax=[]  NCopyOutDataTypeStr=Inherit: Inherit via back propagation  NCopyOutMin=[]  NCopyOutMax=[]  IntegratorContinuousStateAttributes=''  IntegratorStateMustResolveToSignalObject=off  IntegratorRTWStateStorageClass=Auto  FilterContinuousStateAttributes=''  FilterStateMustResolveToSignalObject=off  FilterRTWStateStorageClass=Auto  ParallelPVariant=InternalParameters  IdealPVariant=Disabled  IVariant=InternalParameters  DVariant=InternalParameters  IntegratorVariant=Continuous  SatVariant=Disabled  AWVariant=Passthrough  PCopyVariant=Disabled  TRVariant=Disabled  FdbkBlocksVariant=Forward  IdealPFdbkVariant=Disabled  SatFdbkVariant=Disabled  DerivativeFilterVariant=ContFilter  NVariant=InternalParameters  NCopyVariant=Disabled  FilterICVariant=InternalICsFilter  IntegratorICVariant=InternalICs  ExternalResetVariant=Disabled  TRSumVariant=Passthrough  SumFdbkVariant=Disabled  SumVariant=Sum_PID  TsampFilterVariant=InternalTs  TsampNgainVariant=Passthrough  TsampIntegralVariant=Disabled_SignalSpec  ExternalSaturationOutDataTypeStr=Inherit: Same as second input
  Subtract : Sum  Inputs=-+
  Out1 : Outport
  wires:
  Speed/1 -> Subtract/1
  PID Controller/1 -> Out1/1  "Control Signal"
  Target Speed/1 -> Subtract/2  "Desired Speed"
  Subtract/1 -> PID Controller/1  "Error"

== system Car/Control/old/If Action Subsystem1 ==
  In1 : Inport
  Action Port : ActionPort  ActionPortLabel=else
  Out1 : Outport
  wires:
  In1/1 -> Out1/1

== system Car/Forces/Brakes/If Action Subsystem ==
  In1 : Inport
  Action Port : ActionPort  ActionPortLabel=else
  Out1 : Outport
  wires:
  In1/1 -> Out1/1

== system Car/Forces/Brakes/If Action Subsystem1 ==
  TargetSpeed : Inport
  Action Port : ActionPort  ActionPortLabel=if(u1)
  PID Controller : slpidlib/PID Controller  Controller=PID  Form=Parallel  TimeDomain=Continuous-time  UseExternalTs=off  SampleTime=-1  IntegratorMethod=Forward Euler  FilterMethod=Forward Euler  ControllerParametersSource=internal  P=10  I=1  UseKiTs=off  D=0.5  UseExternalDerivativeSource=off  N=100  UseFilter=on  TunerSelectOption=Transfer Function Based (PID Tuner App)  InitialConditionSource=internal  InitialConditionForIntegrator=0  InitialConditionForFilter=0  DifferentiatorICPrevScaledInput=0  ExternalReset=none  TrackingMode=off  Kt=1  LimitOutput=off  SatLimitsSource=internal  UpperSaturationLimit=inf  LowerSaturationLimit=-inf  LinearizeAsGain=on  AntiWindupMode=none  Kb=1  LimitIntegrator=off  UpperIntegratorSaturationLimit=inf  LowerIntegratorSaturationLimit=-inf  POutMin=[]  POutMax=[]  IOutMin=[]  IOutMax=[]  DOutMin=[]  DOutMax=[]  NOutMin=[]  NOutMax=[]  SumOutMin=[]  SumOutMax=[]  SaturationOutMin=[]  SaturationOutMax=[]  PParamMin=[]  PParamMax=[]  IParamMin=[]  IParamMax=[]  DParamMin=[]  DParamMax=[]  NParamMin=[]  NParamMax=[]  KbParamMin=[]  KbParamMax=[]  KtParamMin=[]  KtParamMax=[]  KbOutMin=[]  KbOutMax=[]  KtOutMin=[]  KtOutMax=[]  IntegratorOutMin=[]  IntegratorOutMax=[]  FilterOutMin=[]  FilterOutMax=[]  SumI1OutMin=[]  SumI1OutMax=[]  SumI2OutMin=[]  SumI2OutMax=[]  SumI3OutMin=[]  SumI3OutMax=[]  SumI4OutMin=[]  SumI4OutMax=[]  SumDOutMin=[]  SumDOutMax=[]  DifferentiatorOutMin=[]  DifferentiatorOutMax=[]  FilterDiffOutCoefMin=[]  FilterDiffOutCoefMax=[]  ReciprocalOutMin=[]  ReciprocalOutMax=[]  SumDenOutMin=[]  SumDenOutMax=[]  SumNumOutMin=[]  SumNumOutMax=[]  DivideOutMin=[]  DivideOutMax=[]  UdiffTsProdOutMin=[]  UdiffTsProdOutMax=[]  NTsProdOutMin=[]  NTsProdOutMax=[]  UintegralTsProdOutMin=[]  UintegralTsProdOutMax=[]  UngainTsProdOutMin=[]  UngainTsProdOutMax=[]  ClampingZeroOutDataTypeStr=Inherit: Inherit via back propagation  ClampingZeroOutMin=[]  ClampingZeroOutMax=[]  FilterDenConstantOutDataTypeStr=Inherit: Inherit via back propagation  FilterDenConstantOutMin=[]  FilterDenConstantOutMax=[]  PCopyOutDataTypeStr=Inherit: Inherit via back propagation  PCopyOutMin=[]  PCopyOutMax=[]  NCopyOutDataTypeStr=Inherit: Inherit via back propagation  NCopyOutMin=[]  NCopyOutMax=[]  IntegratorContinuousStateAttributes=''  IntegratorStateMustResolveToSignalObject=off  IntegratorRTWStateStorageClass=Auto  FilterContinuousStateAttributes=''  FilterStateMustResolveToSignalObject=off  FilterRTWStateStorageClass=Auto  ParallelPVariant=InternalParameters  IdealPVariant=Disabled  IVariant=InternalParameters  DVariant=InternalParameters  IntegratorVariant=Continuous  SatVariant=Disabled  AWVariant=Passthrough  PCopyVariant=Disabled  TRVariant=Disabled  FdbkBlocksVariant=Forward  IdealPFdbkVariant=Disabled  SatFdbkVariant=Disabled  DerivativeFilterVariant=ContFilter  NVariant=InternalParameters  NCopyVariant=Disabled  FilterICVariant=InternalICsFilter  IntegratorICVariant=InternalICs  ExternalResetVariant=Disabled  TRSumVariant=Passthrough  SumFdbkVariant=Disabled  SumVariant=Sum_PID  TsampFilterVariant=InternalTs  TsampNgainVariant=Passthrough  TsampIntegralVariant=Disabled_SignalSpec  ExternalSaturationOutDataTypeStr=Inherit: Same as second input  DerivativeSourceVariant=ErrorSignal  PreIntVariant=InternalPreInt
  brakeForce : Outport
  wires:
  TargetSpeed/1 -> PID Controller/1
  PID Controller/1 -> brakeForce/1

== system Car/Forces/Brakes/If Action Subsystem2 ==
  In1 : Inport
  Action Port : ActionPort  ActionPortLabel=if(u1)
  Out1 : Outport
  wires:
  In1/1 -> Out1/1

== system Car/Forces/Brakes/If Action Subsystem3 ==
  Speed : Inport
  Action Port : ActionPort  ActionPortLabel=else
  Out1 : Outport
  wires:
  Speed/1 -> Out1/1

== system Car/Forces/Propulsion (Motor)/Curent Cap ==
  note: Compare currents and ensure max is not exceeded
  Current : Inport
  RPM : Inport  Port=2
  PowerMode : Inport  Port=3
  Abs : Abs  ZeroCross=off  SaturateOnIntegerOverflow=off
  If : If  IfExpression=u1 ~= 1
  Merge : Merge
  Min : MinMax  Inputs=2
  lookup maximum eco mode current : Subsystem  TreatAsAtomicUnit=on
  lookup maximum power mode current : Subsystem  TreatAsAtomicUnit=on
  current : Outport
  wires:
  PowerMode/1 -> If/1
  If/1 -> lookup maximum eco mode current/Action  "Eco Mode"
  If/2 -> lookup maximum power mode current/Action  "Power Mode"
  RPM/1 -> lookup maximum power mode current/1(RPM), lookup maximum eco mode current/1(RPM)
  lookup maximum eco mode current/1(MaxCurrentEco) -> Merge/1
  lookup maximum power mode current/1(MaxCurrentPower) -> Merge/2
  Merge/1 -> Min/2  "maxCurrent"
  Current/1 -> Abs/1
  Abs/1 -> Min/1
  Min/1 -> current/1

== system Car/Forces/Propulsion (Motor)/Max Torque ==
  In1 : Inport
  Action Port : ActionPort  ActionPortLabel=elseif(..)
  Out1 : Outport
  wires:
  In1/1 -> Out1/1

== system Car/Forces/Propulsion (Motor)/No Torque ==
  In1 : Inport
  Action Port : ActionPort  ActionPortLabel=if(u1 <= MIN_CURRENT)
  Out1 : Outport
  wires:
  In1/1 -> Out1/1

== system Car/Forces/Propulsion (Motor)/Torque Production ==
  Current : Inport
  PowerMode : Inport  Port=2
  If Action Subsystem : Subsystem  TreatAsAtomicUnit=on
  If Action Subsystem1 : Subsystem  TreatAsAtomicUnit=on
  If1 : If  IfExpression=u1 ~= 1
  Merge : Merge
  torque : Outport
  wires:
  Merge/1 -> torque/1  "torque"
  If Action Subsystem/1(torqueEco) -> Merge/1
  If1/2 -> If Action Subsystem1/Action  "Power Mode"
  If1/1 -> If Action Subsystem/Action  "Eco Mode"
  PowerMode/1 -> If1/1
  Current/1 -> If Action Subsystem1/1(current), If Action Subsystem/1(current)
  If Action Subsystem1/1(torqueEco) -> Merge/2

== system Car/Forces/Propulsion (Motor)/Uses Interpolated Data ==
  Current (Signal) : Inport
  Action Port : ActionPort  ActionPortLabel=else
  1-D Lookup Table : Lookup_n-D  NumberOfTableDimensions=1  LookupTableObject=''  BreakpointsForDimension1=INT_CURRENTS  BreakpointsForDimension1FirstPoint=10  BreakpointsForDimension2FirstPoint=10  BreakpointsForDimension1Spacing=12  BreakpointsForDimension2Spacing=12  Table=INT_TORQUES_ECO  DiagnosticForOutOfRangeInput=Warning  InternalRulePriority=Speed  RndMeth=Simplest
  Out1 : Outport
  wires:
  Current (Signal)/1 -> 1-D Lookup Table/1
  1-D Lookup Table/1 -> Out1/1

== system Car/Forces/Resistive Forces/Drag ==
  note: Further thoughts suggest that we may want to find the drag coefficent as a function of the reynolds number instead of the speed.
  note: $C_d \rightarrow C_d(u)$
  note: Find the velocity dependence of the drag coefficient. Effectively we want to transform
  note: $\rho = \text{Air density} \qquad \text{(Setup.m)} \\ A = \text{Vehicle frontal area} \qquad \text{(Setup.m)} \\ C_d = \text{Vehicle drag coefficient} \qquad \text{(Calculated)} \\ u = \text{Vehicle speed} \qquad \text{(Subsystem Input)}$
  note: Where,
  note: $F_D = \frac{1}{2} \rho A C_d u^2$
  note: This computes the drag force on the vehicle due to motion using the formula
  note: To Do:
  note: Drag Force
  Velocity : Inport
  0.5 rho A : Gain  Gain=0.5 * AIR_DENSITY * FRONTAL_AREA
  Drag Coefficient : Gain  Gain=DRAG_COEFFICIENT
  Square : Math  Operator=square
  Drag Force : Outport
  wires:
  Velocity/1 -> Square/1  "[m / s]"
  Square/1 -> 0.5 rho A/1  "[m^2/s^2]"
  0.5 rho A/1 -> Drag Coefficient/1  "[N]"
  Drag Coefficient/1 -> Drag Force/1  "[N]"

== system Car/Forces/Resistive Forces/Rolling Resistance ==
  note: This computes the rolling resitance on the vehicle due to motion using the formula
  note: To Do:
  note: $C_{RR} = \text{Coefficient of Rolling Resistance \quad (Reddit)} \\ N = \text{Normal Force \quad (Weight)}$
  note: Where,
  note: Find the velocity dependence of the rolling resistance coefficient. Effectively we want to transform
      | Account for elevation changes
  note: Rolling Resistance
  note: $F_{RR} = C_{RR} N$
  Velocity : Inport
  Normal Force : Inport  Port=2
  Constant : Constant  Value=C_ROLLING_RESISTANCE
  Product : Product
  Rolling Resistance : Outport
  wires:
  Velocity/1 -> ?
  Constant/1 -> Product/1  "[-]"
  Product/1 -> Rolling Resistance/1  "[N]"
  Normal Force/1 -> Product/2  "[N]"

== system Car/Control/Filter if below min SOC/Control Mode/Power Control ==
  power : Inport
  target power : Inport  Port=2
  Action Port : ActionPort  ActionPortLabel=else
  PID Controller : slpidlib/PID Controller  Controller=PID  Form=Parallel  TimeDomain=Continuous-time  UseExternalTs=off  SampleTime=-1  IntegratorMethod=Forward Euler  FilterMethod=Forward Euler  ControllerParametersSource=internal  P=P_POWER  I=I_POWER  UseKiTs=off  D=D_POWER  UseExternalDerivativeSource=off  N=100  UseFilter=on  TunerSelectOption=Transfer Function Based (PID Tuner App)  InitialConditionSource=internal  InitialConditionForIntegrator=0  InitialConditionForFilter=0  DifferentiatorICPrevScaledInput=0  ExternalReset=none  TrackingMode=off  Kt=1  LimitOutput=off  SatLimitsSource=internal  UpperSaturationLimit=inf  LowerSaturationLimit=-inf  LinearizeAsGain=on  AntiWindupMode=none  Kb=1  LimitIntegrator=off  UpperIntegratorSaturationLimit=inf  LowerIntegratorSaturationLimit=-inf  POutMin=[]  POutMax=[]  IOutMin=[]  IOutMax=[]  DOutMin=[]  DOutMax=[]  NOutMin=[]  NOutMax=[]  SumOutMin=[]  SumOutMax=[]  SaturationOutMin=[]  SaturationOutMax=[]  PParamMin=[]  PParamMax=[]  IParamMin=[]  IParamMax=[]  DParamMin=[]  DParamMax=[]  NParamMin=[]  NParamMax=[]  KbParamMin=[]  KbParamMax=[]  KtParamMin=[]  KtParamMax=[]  KbOutMin=[]  KbOutMax=[]  KtOutMin=[]  KtOutMax=[]  IntegratorOutMin=[]  IntegratorOutMax=[]  FilterOutMin=[]  FilterOutMax=[]  SumI1OutMin=[]  SumI1OutMax=[]  SumI2OutMin=[]  SumI2OutMax=[]  SumI3OutMin=[]  SumI3OutMax=[]  SumI4OutMin=[]  SumI4OutMax=[]  SumDOutMin=[]  SumDOutMax=[]  DifferentiatorOutMin=[]  DifferentiatorOutMax=[]  FilterDiffOutCoefMin=[]  FilterDiffOutCoefMax=[]  ReciprocalOutMin=[]  ReciprocalOutMax=[]  SumDenOutMin=[]  SumDenOutMax=[]  SumNumOutMin=[]  SumNumOutMax=[]  DivideOutMin=[]  DivideOutMax=[]  UdiffTsProdOutMin=[]  UdiffTsProdOutMax=[]  NTsProdOutMin=[]  NTsProdOutMax=[]  UintegralTsProdOutMin=[]  UintegralTsProdOutMax=[]  UngainTsProdOutMin=[]  UngainTsProdOutMax=[]  ClampingZeroOutDataTypeStr=Inherit: Inherit via back propagation  ClampingZeroOutMin=[]  ClampingZeroOutMax=[]  FilterDenConstantOutDataTypeStr=Inherit: Inherit via back propagation  FilterDenConstantOutMin=[]  FilterDenConstantOutMax=[]  PCopyOutDataTypeStr=Inherit: Inherit via back propagation  PCopyOutMin=[]  PCopyOutMax=[]  NCopyOutDataTypeStr=Inherit: Inherit via back propagation  NCopyOutMin=[]  NCopyOutMax=[]  IntegratorContinuousStateAttributes=''  IntegratorStateMustResolveToSignalObject=off  IntegratorRTWStateStorageClass=Auto  FilterContinuousStateAttributes=''  FilterStateMustResolveToSignalObject=off  FilterRTWStateStorageClass=Auto  ParallelPVariant=InternalParameters  IdealPVariant=Disabled  IVariant=InternalParameters  DVariant=InternalParameters  IntegratorVariant=Continuous  SatVariant=Disabled  AWVariant=Passthrough  PCopyVariant=Disabled  TRVariant=Disabled  FdbkBlocksVariant=Forward  IdealPFdbkVariant=Disabled  SatFdbkVariant=Disabled  DerivativeFilterVariant=ContFilter  NVariant=InternalParameters  NCopyVariant=Disabled  FilterICVariant=InternalICsFilter  IntegratorICVariant=InternalICs  ExternalResetVariant=Disabled  TRSumVariant=Passthrough  SumFdbkVariant=Disabled  SumVariant=Sum_PID  TsampFilterVariant=InternalTs  TsampNgainVariant=Passthrough  TsampIntegralVariant=Disabled_SignalSpec  ExternalSaturationOutDataTypeStr=Inherit: Same as second input  DerivativeSourceVariant=ErrorSignal  PreIntVariant=InternalPreInt
  Subtract : Sum  Inputs=-+
  Out1 : Outport
  wires:
  power/1 -> Subtract/1
  PID Controller/1 -> Out1/1  "controlPowerSignal"
  Subtract/1 -> PID Controller/1  "powerError"
  target power/1 -> Subtract/2
